simulink model "forward"  (R2020b)
settings: Solver=VariableStepAuto  StartTime=0.0  StopTime=20.0  RelTol=1e-3
values from neighbouring files (symbols this model uses):
  Cvx1 = 182.87    [Calculations.m]
  Cvx2 = 33    [Calculations.m]
  k1_m = (M^2 + M* sqrt(M^2 - 1)) / ( 4 * T_v * K_v)    [Calculations.m]
  k2_m = ( T_propulsion_x*(m+lambda11) - (2*Cvx1 * V_linearization + Cvx2)* T_v^2) /     ( T_v^2 * K_propulsion_x )    (= 5.31997888912)    [Calculations.m]
  K_thruster = P1 / U1    (= 24.525)    [Calculations.m]
  lambda11 = 12.72    [Calculations.m]
  m = 300    [Calculations.m]
  T_thruster = 0.3    [Calculations.m]
settings Model: Creator=corsair  LastModifiedBy=corsair

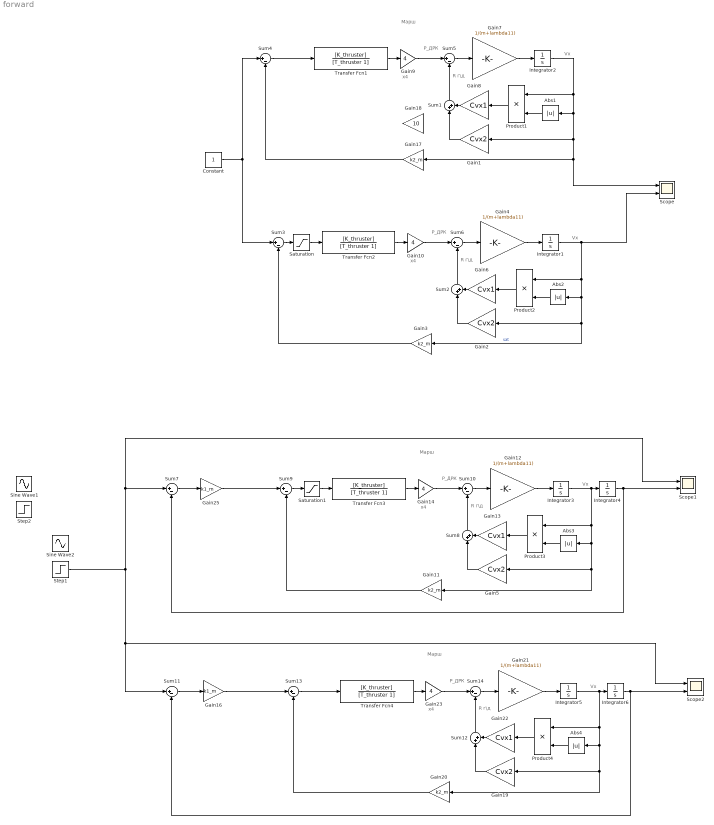
== system forward ==
  note: x4
  note: R г\д
  note: P_ДРК
  note: Марш
  note: Vx
  note: x4
  note: R г\д
  note: P_ДРК
  note: Vx
  note: x4
  note: R г\д
  note: P_ДРК
  note: Марш
  note: Vx
  note: x4
  note: R г\д
  note: P_ДРК
  note: Марш
  note: Vx
  Abs{1..4} (4 alike) : Abs
  Constant : Constant
  Gain{1..2,5,19} (4 alike) : Gain  Gain=Cvx2
  Gain{9..10,14,23} (4 alike) : Gain  Gain=4
  Gain{3,11,17,20} (4 alike) : Gain  Gain=k2_m
  Gain{4,7,12,21} (4 alike) : Gain  Gain=1/(m+lambda11)
  Gain{6,8,13,22} (4 alike) : Gain  Gain=Cvx1
  Gain16 : Gain  Gain=k1_m
  Gain18 : Gain  Gain=10
  Gain25 : Gain  Gain=k1_m
  Integrator{1..6} (6 alike) : Integrator
  Product{1..4} (4 alike) : Product
  Saturation : Saturate
  Saturation1 : Saturate
  Scope : Scope  NumInputPorts=2
  Scope1 : Scope  NumInputPorts=2
  Scope2 : Scope  NumInputPorts=2
  Sine Wave1 : Sin  SampleTime=0
  Sine Wave2 : Sin  SampleTime=0
  Step1 : Step  SampleTime=0
  Step2 : Step  SampleTime=0
  Sum{1..2,8,12} (4 alike) : Sum  Inputs=|++
  Sum{3..7,9..11,13..14} (10 alike) : Sum  Inputs=|+-
  Transfer Fcn{1..4} (4 alike) : TransferFcn  Numerator=[K_thruster]  Denominator=[T_thruster 1]
  wires:
  Abs1/1 -> Product1/2
  Gain9/1 -> Sum5/1
  Integrator2/1 -> Gain17/1, Scope/1, Gain1/1, Abs1/1, Product1/1
  Gain7/1 -> Integrator2/1
  Sum5/1 -> Gain7/1
  Sum4/1 -> Transfer Fcn1/1
  Transfer Fcn1/1 -> Gain9/1
  Gain17/1 -> Sum4/2
  Product1/1 -> Gain8/1
  Gain8/1 -> Sum1/2
  Sum1/1 -> Sum5/2
  Gain1/1 -> Sum1/1
  Gain2/1 -> Sum2/1
  Sum2/1 -> Sum6/2
  Gain6/1 -> Sum2/2
  Product2/1 -> Gain6/1
  Gain3/1 -> Sum3/2
  Transfer Fcn2/1 -> Gain10/1
  Sum3/1 -> Saturation/1
  Sum6/1 -> Gain4/1
  Gain4/1 -> Integrator1/1
  Constant/1 -> Sum4/1, Sum3/1
  Integrator1/1 -> Product2/1, Abs2/1, Gain3/1, Gain2/1, Scope/2  "sat"
  Gain10/1 -> Sum6/1
  Abs2/1 -> Product2/2
  Saturation/1 -> Transfer Fcn2/1
  Integrator6/1 -> Sum11/2, Scope2/2
  Sum13/1 -> Transfer Fcn4/1
  Gain16/1 -> Sum13/1
  Abs4/1 -> Product4/2
  Gain23/1 -> Sum14/1
  Integrator5/1 -> Integrator6/1, Gain20/1, Gain19/1, Abs4/1, Product4/1
  Gain21/1 -> Integrator5/1
  Sum14/1 -> Gain21/1
  Transfer Fcn4/1 -> Gain23/1
  Gain20/1 -> Sum13/2
  Product4/1 -> Gain22/1
  Gain22/1 -> Sum12/2
  Sum12/1 -> Sum14/2
  Gain19/1 -> Sum12/1
  Step1/1 -> Sum11/1, Scope2/1, Sum7/1, Scope1/1
  Gain5/1 -> Sum8/1
  Sum8/1 -> Sum10/2
  Gain13/1 -> Sum8/2
  Product3/1 -> Gain13/1
  Gain11/1 -> Sum9/2
  Transfer Fcn3/1 -> Gain14/1
  Sum10/1 -> Gain12/1
  Gain12/1 -> Integrator3/1
  Integrator3/1 -> Product3/1, Abs3/1, Gain5/1, Gain11/1, Integrator4/1
  Gain14/1 -> Sum10/1
  Abs3/1 -> Product3/2
  Gain25/1 -> Sum9/1
  Sum9/1 -> Saturation1/1
  Integrator4/1 -> Scope1/2, Sum7/2
  Saturation1/1 -> Transfer Fcn3/1
  Sum7/1 -> Gain25/1
  Sum11/1 -> Gain16/1
